simulink model "ModelGreenhouse"  (R2018a)
settings: Solver=FixedStepAuto  StartTime=0  StopTime=432000  FixedStep=5  RelTol=1e-1
undefined symbols (not defined in the file or in its folder): magnitude
libraries: simulink x6
(part 3 of 3)

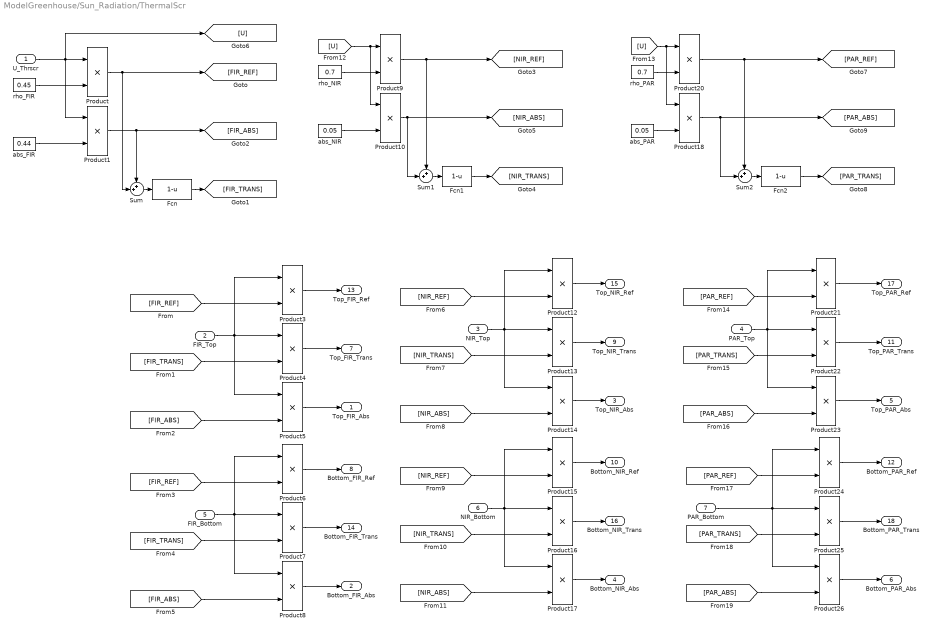
== system ModelGreenhouse/Sun_Radiation/ThermalScr ==
  U_Thrscr : Inport
  FIR_Top : Inport  Port=2
  NIR_Top : Inport  Port=3
  PAR_Top : Inport  Port=4
  FIR_Bottom : Inport  Port=5
  NIR_Bottom : Inport  Port=6
  PAR_Bottom : Inport  Port=7
  Fcn : Fcn  Expr=1-u
  Fcn1 : Fcn  Expr=1-u
  Fcn2 : Fcn  Expr=1-u
  Product{,1,3..10,12..18,20..26} (24 alike) : Product
  Sum : Sum  Inputs=++|
  Sum1 : Sum  Inputs=++|
  Sum2 : Sum  Inputs=++|
  abs_FIR : Constant  Value=0.44
  abs_NIR : Constant  Value=0.05
  abs_PAR : Constant  Value=0.05
  rho_FIR : Constant  Value=0.45
  rho_NIR : Constant  Value=0.7
  rho_PAR : Constant  Value=0.7
  Top_FIR_Abs : Outport
  Bottom_FIR_Abs : Outport  Port=2
  Top_NIR_Abs : Outport  Port=3
  Bottom_NIR_Abs : Outport  Port=4
  Top_PAR_Abs : Outport  Port=5
  Bottom_PAR_Abs : Outport  Port=6
  Top_FIR_Trans : Outport  Port=7
  Bottom_FIR_Ref : Outport  Port=8
  Top_NIR_Trans : Outport  Port=9
  Bottom_NIR_Ref : Outport  Port=10
  Top_PAR_Trans : Outport  Port=11
  Bottom_PAR_Ref : Outport  Port=12
  Top_FIR_Ref : Outport  Port=13
  Bottom_FIR_Trans : Outport  Port=14
  Top_NIR_Ref : Outport  Port=15
  Bottom_NIR_Trans : Outport  Port=16
  Top_PAR_Ref : Outport  Port=17
  Bottom_PAR_Trans : Outport  Port=18
  wires:
  FIR_Top/1 -> Product3/1, Product5/1, Product4/1
  abs_FIR/1 -> Product1/2
  U_Thrscr/1 -> Product1/1, Product/1, [U]
  Fcn/1 -> [FIR_TRANS]
  rho_FIR/1 -> Product/2
  Sum/1 -> Fcn/1
  Product/1 -> Sum/2, [FIR_REF]
  [FIR_REF] -> Product3/2
  Product4/1 -> Top_FIR_Trans/1
  Product3/1 -> Top_FIR_Ref/1
  Product6/1 -> Bottom_FIR_Ref/1
  Product7/1 -> Bottom_FIR_Trans/1
  Product5/1 -> Top_FIR_Abs/1
  Product8/1 -> Bottom_FIR_Abs/1
  [FIR_ABS] -> Product5/2
  [FIR_TRANS] -> Product4/2
  [FIR_TRANS] -> Product7/2
  [FIR_ABS] -> Product8/2
  FIR_Bottom/1 -> Product6/1, Product8/1, Product7/1
  [FIR_REF] -> Product6/2
  abs_NIR/1 -> Product10/2
  rho_NIR/1 -> Product9/2
  Sum1/1 -> Fcn1/1
  Product9/1 -> Sum1/1, [NIR_REF]
  [NIR_TRANS] -> Product13/2
  [NIR_REF] -> Product12/2
  NIR_Top/1 -> Product12/1, Product14/1, Product13/1
  [NIR_ABS] -> Product14/2
  [NIR_REF] -> Product15/2
  [NIR_ABS] -> Product17/2
  [NIR_TRANS] -> Product16/2
  NIR_Bottom/1 -> Product15/1, Product17/1, Product16/1
  Product14/1 -> Top_NIR_Abs/1
  Product13/1 -> Top_NIR_Trans/1
  Product12/1 -> Top_NIR_Ref/1
  Product15/1 -> Bottom_NIR_Ref/1
  Product16/1 -> Bottom_NIR_Trans/1
  Product17/1 -> Bottom_NIR_Abs/1
  [U] -> Product10/1, Product9/1
  [U] -> Product18/1, Product20/1
  Sum2/1 -> Fcn2/1
  rho_PAR/1 -> Product20/2
  abs_PAR/1 -> Product18/2
  [PAR_REF] -> Product21/2
  PAR_Top/1 -> Product21/1, Product23/1, Product22/1
  [PAR_TRANS] -> Product22/2
  [PAR_ABS] -> Product23/2
  Product21/1 -> Top_PAR_Ref/1
  Product22/1 -> Top_PAR_Trans/1
  Product23/1 -> Top_PAR_Abs/1
  Product26/1 -> Bottom_PAR_Abs/1
  [PAR_ABS] -> Product26/2
  [PAR_REF] -> Product24/2
  [PAR_TRANS] -> Product25/2
  Product24/1 -> Bottom_PAR_Ref/1
  Product25/1 -> Bottom_PAR_Trans/1
  PAR_Bottom/1 -> Product24/1, Product26/1, Product25/1
  Product1/1 -> Sum/1, [FIR_ABS]
  Product10/1 -> [NIR_ABS], Sum1/2
  Fcn1/1 -> [NIR_TRANS]
  Fcn2/1 -> [PAR_TRANS]
  Product18/1 -> Sum2/2, [PAR_ABS]
  Product20/1 -> Sum2/1, [PAR_REF]

== system ModelGreenhouse/Sun_Radiation/floor ==
  FIR_Top : Inport
  NIR_Top : Inport  Port=2
  PAR_Top : Inport  Port=3
  alpha_FIR : Gain
  alpha_NIR : Gain  Gain=0.5
  alpha_PAR : Gain  Gain=0.35
  rho_FIR : Gain  Gain=0
  rho_NIR : Gain  Gain=0.5
  rho_PAR : Gain  Gain=0.65
  tau_FIR : Gain  Gain=0
  tau_NIR : Gain  Gain=0
  tau_PAR : Gain  Gain=0
  Top_FIR_Abs : Outport
  Top_NIR_Abs : Outport  Port=2
  Top_PAR_Abs : Outport  Port=3
  Top_FIR_Ref : Outport  Port=4
  Top_NIR_Ref : Outport  Port=5
  Top_PAR_Ref : Outport  Port=6
  Top_FIR_Trans : Outport  Port=7
  Top_NIR_Trans : Outport  Port=8
  Top_PAR_Trans : Outport  Port=9
  wires:
  tau_FIR/1 -> Top_FIR_Trans/1
  rho_FIR/1 -> Top_FIR_Ref/1
  FIR_Top/1 -> tau_FIR/1, alpha_FIR/1, rho_FIR/1
  alpha_FIR/1 -> Top_FIR_Abs/1
  rho_NIR/1 -> Top_NIR_Ref/1
  tau_NIR/1 -> Top_NIR_Trans/1
  NIR_Top/1 -> tau_NIR/1, rho_NIR/1, alpha_NIR/1
  alpha_NIR/1 -> Top_NIR_Abs/1
  tau_PAR/1 -> Top_PAR_Trans/1
  rho_PAR/1 -> Top_PAR_Ref/1
  alpha_PAR/1 -> Top_PAR_Abs/1
  PAR_Top/1 -> tau_PAR/1, alpha_PAR/1, rho_PAR/1

== system ModelGreenhouse/Plants(transpiration)/Stomatal Resistance /CO2 plenaty factor ==
  C_CO2 : Inport
  I_d/n : Inport  Port=2
  I_A_can : Inport  Port=3
  Bias6 : Bias  Bias=-200
  Bias7 : Bias  Bias=1
  Bias8 : Bias  Bias=1
  Gain5 : Gain  Gain=6.08e-7
  Gain6 : Gain  Gain=1.1e-11
  MATLAB Function1 : MATLAB Function  TreatAsAtomicUnit=on
  MATLAB Function2 : MATLAB Function  TreatAsAtomicUnit=on
  Math Function3 : Math  Operator=magnitude^2  SaturateOnIntegerOverflow=on
  max : Constant  Value=1.49
  max_CO2 : Constant  Value=1100
  f(C_CO2) : Outport
  wires:
  Math Function3/1 -> Gain6/1, Gain5/1
  MATLAB Function1/1(Out) -> MATLAB Function2/2(u_lower)
  C_CO2/1 -> MATLAB Function2/4(key), Bias6/1
  max/1 -> MATLAB Function2/1(u_upper)
  Gain6/1 -> Bias8/1
  I_A_can/1 -> MATLAB Function1/4(key)
  Gain5/1 -> Bias7/1
  Bias8/1 -> MATLAB Function1/2(u_lower)
  max_CO2/1 -> MATLAB Function2/3(thres)
  Bias6/1 -> Math Function3/1
  Bias7/1 -> MATLAB Function1/1(u_upper)
  I_d/n/1 -> MATLAB Function1/3(thres)
  MATLAB Function2/1(Out) -> f(C_CO2)/1  "f(C_CO2)"

== system ModelGreenhouse/Plants(transpiration)/Stomatal Resistance /Radiation plenaty facor ==
  PAR : Inport
  LAI : Inport  Port=2
  Bias : Bias  Bias=4.3
  Bias1 : Bias  Bias=0.54
  Divide2 : Product  Inputs=*/
  Divide3 : Product  Inputs=*/
  Gain2 : Gain  Gain=2
  f(I_sun) : Outport
  wires:
  Bias1/1 -> Divide3/2
  Gain2/1 -> Divide2/2
  LAI/1 -> Gain2/1
  Divide2/1 -> Bias/1, Bias1/1
  Bias/1 -> Divide3/1
  Divide3/1 -> f(I_sun)/1  "f(I_sun)"
  PAR/1 -> Divide2/1

== system ModelGreenhouse/Plants(transpiration)/Stomatal Resistance /Subsystem ==
  I_d/n : Inport
  I_A_can : Inport  Port=2
  VP : Inport  Port=3
  VP_S : Inport  Port=4
  Fcn4 : Fcn  Expr=4.3e-6 * u +1
  Fcn5 : Fcn  Expr=5.2e-6 * u +1
  MATLAB Function3 : MATLAB Function  TreatAsAtomicUnit=on
  Math Function4 : Math  Operator=magnitude^2  SaturateOnIntegerOverflow=on
  Saturation : Saturate  UpperLimit=3.9
  Sum2 : Sum  Inputs=|+-
  f(C_H2O) : Outport
  wires:
  I_A_can/1 -> MATLAB Function3/4(key)
  Fcn5/1 -> MATLAB Function3/2(u_lower)
  Saturation/1 -> f(C_H2O)/1  "f(C_H2O)"
  Math Function4/1 -> Fcn5/1, Fcn4/1
  Sum2/1 -> Math Function4/1
  Fcn4/1 -> MATLAB Function3/1(u_upper)
  MATLAB Function3/1(Out) -> Saturation/1
  VP/1 -> Sum2/1
  VP_S/1 -> Sum2/2
  I_d/n/1 -> MATLAB Function3/3(thres)

== system ModelGreenhouse/Plants(transpiration)/Stomatal Resistance /Temperature Plenaty factor ==
  T_can : Inport
  I_d/n : Inport  Port=2
  I_A_can : Inport  Port=3
  Bias2 : Bias  Bias=-33.6
  Bias3 : Bias  Bias=1
  Bias4 : Bias  Bias=-24.512
  Bias5 : Bias  Bias=1
  Gain3 : Gain  Gain=0.5e-2
  Gain4 : Gain  Gain=2.2593e-2
  MATLAB Function : MATLAB Function  TreatAsAtomicUnit=on
  Math Function1 : Math  Operator=magnitude^2  SaturateOnIntegerOverflow=on
  Math Function2 : Math  Operator=magnitude^2  SaturateOnIntegerOverflow=on
  f(Tcan) : Outport
  wires:
  Bias4/1 -> Math Function2/1
  Bias2/1 -> Math Function1/1
  Gain4/1 -> Bias5/1
  Math Function1/1 -> Gain3/1
  Bias3/1 -> MATLAB Function/2(u_lower)
  T_can/1 -> Bias2/1, Bias4/1
  Math Function2/1 -> Gain4/1
  Gain3/1 -> Bias3/1
  Bias5/1 -> MATLAB Function/1(u_upper)
  I_d/n/1 -> MATLAB Function/3(thres)
  I_A_can/1 -> MATLAB Function/4(key)
  MATLAB Function/1(Out) -> f(Tcan)/1  "f(Tcan)"

== matlab function ModelGreenhouse/Plants(transpiration)/Stomatal Resistance /CO2 plenaty factor/MATLAB Function1 ==
  data: u_upper input; Out output; u_lower input; thres input; key input
function Out = Smoothing(u_upper,u_lower,thres,key)
    SFL = 1/(1 + exp( 50 * (key - thres)));
    SFH = 1/(1 + exp( -50 * (key - thres)));
    Out = u_upper * SFH + u_lower * SFL;
end

== matlab function ModelGreenhouse/Plants(transpiration)/Stomatal Resistance /Temperature Plenaty factor/MATLAB Function ==
  data: u_upper input; Out output; u_lower input; thres input; key input
function Out = Smoothing(u_upper,u_lower,thres,key)
    SFL = 1/(1 + exp( 50 * (key - thres)));
    SFH = 1/(1 + exp( -50 * (key - thres)));
    Out = u_upper * SFH + u_lower * SFL;
end

== matlab function ModelGreenhouse/Plants(transpiration)/Stomatal Resistance /CO2 plenaty factor/MATLAB Function2 ==
  data: u_upper input; Out output; u_lower input; thres input; key input
function Out = Smoothing(u_upper,u_lower,thres,key)
    SFL = 1/(1 + exp( 50 * (key - thres)));
    SFH = 1/(1 + exp( -50 * (key - thres)));
    Out = u_upper * SFH + u_lower * SFL;
end

== matlab function ModelGreenhouse/Plants(transpiration)/Stomatal Resistance /Subsystem/MATLAB Function3 ==
  data: u_upper input; Out output; u_lower input; thres input; key input
function Out = Smoothing(u_upper,u_lower,thres,key)
    SFL = 1/(1 + exp( 50 * (key - thres)));
    SFH = 1/(1 + exp( -50 * (key - thres)));
    Out = u_upper * SFH + u_lower * SFL;
end

== matlab function ModelGreenhouse/Plants(transpiration)/MATLAB Function4 ==
  data: u_upper input; Out output; u_lower input; thres input; key input
function Out = Smoothing(u_upper,u_lower,thres,key)
    SFL = 1/(1 + exp( 50 * (key - thres)));
    SFH = 1/(1 + exp( -50 * (key - thres)));
    Out = u_upper * SFH + u_lower * SFL;
    if Out < 0 
        Out = 0;
    end
end

== matlab function ModelGreenhouse/Air -> Floor/MATLAB Function2 ==
  data: u_upper input; Out output; u_lower input; thres input; key input
function Out = Smoothing(u_upper,u_lower,thres,key)
    SFL = 1/(1 + exp( 50 * (key - thres)));
    SFH = 1/(1 + exp( -50 * (key - thres)));
    Out = u_upper * SFH + u_lower * SFL;
end

== matlab function ModelGreenhouse/MATLAB Function ==
  data: Temp input; VP_sat output
function VP_sat = satVP(Temp)
    VP_h = 610.780 * exp(17.08085 * Temp/(234.175 + Temp));
    VP_l = 610.714 * exp(22.44294 * Temp/(272.440 + Temp));
    SF_H = 1/(1 + exp(-50 * Temp));
    SF_L = 1/(1 + exp(50 * Temp));
    VP_sat = VP_h * SF_H + VP_l * SF_L;
end

== matlab function ModelGreenhouse/Cover(out->covout)/MATLAB Function1 ==
  data: u_upper input; Out output; u_lower input; thres input; key input
function Out = Smoothing(u_upper,u_lower,thres,key)
    SFL = 1/(1 + exp( 50 * (key - thres)));
    SFH = 1/(1 + exp( -50 * (key - thres)));
    Out = u_upper * SFH + u_lower * SFL;
end

== matlab function ModelGreenhouse/Cover(Condensation)/MATLAB Function2 ==
  data: u_upper input; Out output; u_lower input; thres input; key input
function Out = Smoothing(u_upper,u_lower,thres,key)
    SFL = 1/(1 + exp( 500 * (key - thres)));
    SFH = 1/(1 + exp( -500 * (key - thres)));
    %Out = u_upper * SFH + u_lower * SFL;
    Out = u_upper * SFH + u_lower * SFL;
    if Out < 0 
        Out = 0;
    end
end

== matlab function ModelGreenhouse/Plants(transpiration)/MATLAB Function5 ==
  data: Temp input; VP_sat output
function VP_sat = satVP(Temp)
    VP_h = 610.780 * exp(17.08085 * Temp/(234.175 + Temp));
    VP_l = 610.714 * exp(22.44294 * Temp/(272.440 + Temp));
    SF_H = 1/(1 + exp(-50 * Temp));
    SF_L = 1/(1 + exp(50 * Temp));
    VP_sat = VP_h * SF_H + VP_l * SF_L;
end

== matlab function ModelGreenhouse/MATLAB Function1 ==
  data: Temp input; VP_sat output
function VP_sat = satVP(Temp)
    VP_h = 610.780 * exp(17.08085 * Temp/(234.175 + Temp));
    VP_l = 610.714 * exp(22.44294 * Temp/(272.440 + Temp));
    SF_H = 1/(1 + exp(-50 * Temp));
    SF_L = 1/(1 + exp(50 * Temp));
    VP_sat = VP_h * SF_H + VP_l * SF_L;
end

== matlab function ModelGreenhouse/ScrU(Condensation)/MATLAB Function2 ==
  data: u_upper input; Out output; u_lower input; thres input; key input
function Out = Smoothing(u_upper,u_lower,thres,key)
    SFL = 1/(1 + exp( 50 * (key - thres)));
    SFH = 1/(1 + exp( -50 * (key - thres)));
    %Out = u_upper * SFH + u_lower * SFL;
    Out = u_upper * SFH + u_lower * SFL;
    if Out < 0 
        Out = 0;
    end
end

== matlab function ModelGreenhouse/ScrB(Condensation)/MATLAB Function2 ==
  data: u_upper input; Out output; u_lower input; thres input; key input
function Out = Smoothing(u_upper,u_lower,thres,key)
    SFL = 1/(1 + exp( 50 * (key - thres)));
    SFH = 1/(1 + exp( -50 * (key - thres)));
    %Out = u_upper * SFH + u_lower * SFL;
    Out = u_upper * SFH + u_lower * SFL;
    if Out < 0 
        Out = 0;
    end
end

== matlab function ModelGreenhouse/RoofStrategy/MATLAB Function ==
  data: T_air input; y output; Tset input
function y = PT(T_air,Tset)
    if Tset - T_air > 5 % Closed it for heating up
        y = 0;
    else
        y =  1 - 0.2 * (Tset - T_air);
        if y > 1
            y = 1;
        end
    end
end

== matlab function ModelGreenhouse/RoofStrategy/MATLAB Function1 ==
  data: RH_air input; y output; RH_out input; RH_set input
function y = PRH(RH_air,RH_out,RH_set)
    if RH_set - RH_air > 10
        y = 0;
    else
        y = 1 - 0.1 * (RH_set - RH_air);
        if y > 1 
            y = 1;
        end
    end
    if RH_out >= RH_air
        y = 0;
    end
end

== matlab function ModelGreenhouse/Fogging/MATLAB Function ==
  data: RH input; U output; RHset input
function U = RHFogging(RH,RHset)
    if RH > RHset 
        U = 0;
    elseif RHset - RH > 10
        U = 1;
    else
        U = 0.1 * (RHset - RH);
    end
end

== matlab function ModelGreenhouse/SideVentControl/MATLAB Function ==
  data: Enable input; y output; Tout input; Tin input; Status input
function y = Enable(Enable,Tout,Tin,Status)
    y = 0;
    if Status == 0
        y = 1;
    elseif Tout < Tin
        y = 1;
    end
    y = Enable * y;
end
